simulink model "harvest"  (R2024b)
settings: Solver=VariableStepAuto  StartTime=0.0  StopTime=100  RelTol=1e-3
settings Model: Creator=Botló  LastModifiedBy=Botló

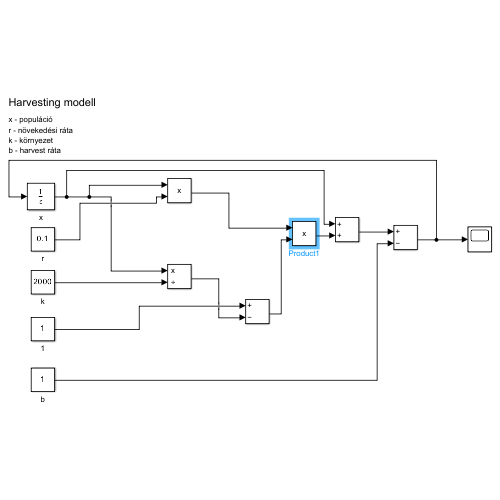
[thumbnail: Simulink's stored preview of the top-level diagram]
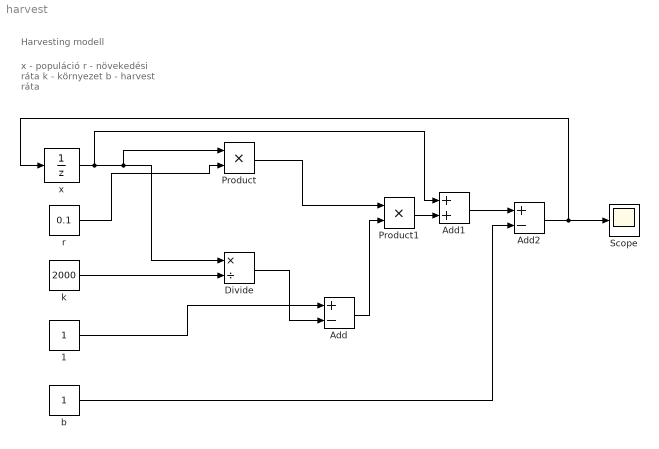
== system harvest ==
  note: Harvesting modell
  note: x - populáció
      | r - növekedési ráta
      | k - környezet
      | b - harvest ráta
  1 : Constant
  Add : Sum  Inputs=+-
  Add1 : Sum
  Add2 : Sum  Inputs=+-
  Divide : Product  Inputs=*/
  Product : Product
  Product1 : Product
  Scope : Scope
  b : Constant
  k : Constant  Value=2000
  r : Constant  Value=0.1
  x : UnitDelay  InitialCondition=100  HasFrameUpgradeWarning=on
  wires:
  r/1 -> Product/2
  x/1 -> Add1/1, Divide/1, Product/1
  k/1 -> Divide/2
  1/1 -> Add/1
  Divide/1 -> Add/2
  Product/1 -> Product1/1
  Add/1 -> Product1/2
  Product1/1 -> Add1/2
  Add1/1 -> Add2/1
  b/1 -> Add2/2
  Add2/1 -> Scope/1, x/1
